simulink subsystem "V"  (R2024a)
settings: Solver=VariableStepAuto  StartTime=0.0  StopTime=10.0  RelTol=1e-3
settings Model: Creator=Dell  LastModifiedBy=mrvol

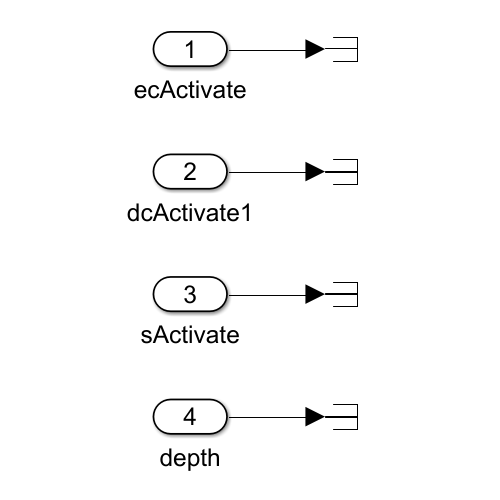
[thumbnail: Simulink's stored preview of the top-level diagram]
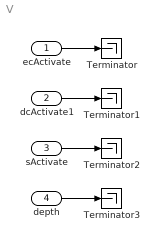
== system V ==
  ecActivate : Inport
  dcActivate1 : Inport  Port=2
  sActivate : Inport  Port=3
  depth : Inport  Port=4
  Terminator{,1..3} (4 alike) : Terminator
  wires:
  ecActivate/1 -> Terminator/1
  dcActivate1/1 -> Terminator1/1
  sActivate/1 -> Terminator2/1
  depth/1 -> Terminator3/1
